simulink model "Open_Loop_No_PLL"  (R2020b)
settings: Solver=ode1  StartTime=0  StopTime=1  FixedStep=Time_Step  MaxStep=100e-6  RelTol=1e-3
undefined symbols (not defined in the file): fb, fn, Ib2, Kp_Rvi_pu, Lc_eq, Lg, Rg, Sb, SCR, Sn, Theta_Vvsc0, Time_Step, Va0, Vb0, Vb1, Vb2, Vc0, Vm0, VSC01_id0, Vvsc0, wb, Zb
libraries: powerlib x23, Control_Lib x22, Source_Lib x3, simulink x2
(part 2 of 2)

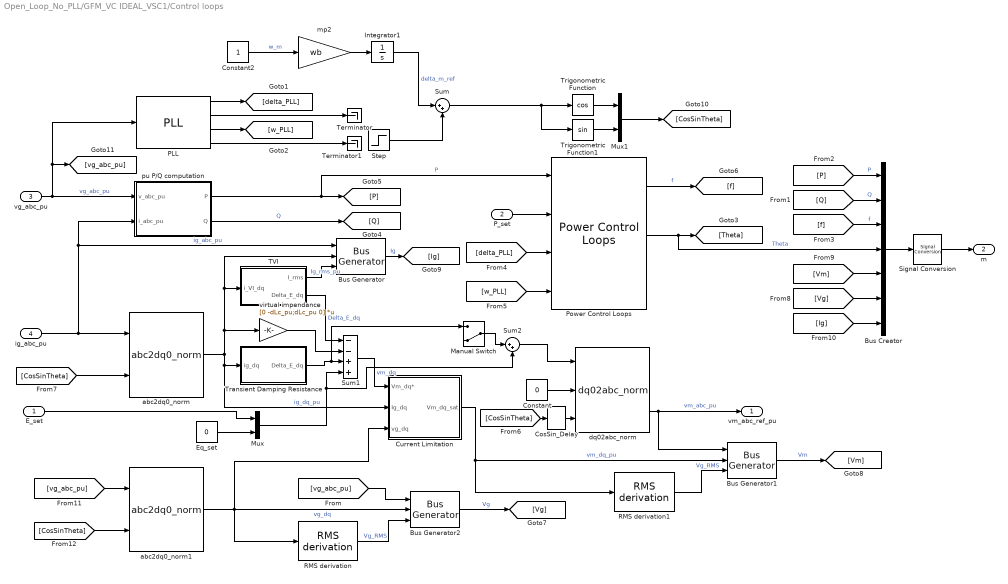
== system Open_Loop_No_PLL/GFM_VC IDEAL_VSC1/Control loops ==
  E_set : Inport
  P_set : Inport  Port=2
  vg_abc_pu : Inport  Port=3
  ig_abc_pu : Inport  Port=4
  " pu P/Q computation" : Subsystem  DialogController=POWERSYS.PowerSysDialog
  Bus Creator : BusCreator  Inputs=7
  Bus Generator : Control_Lib/Bus Generator  Gpu=Ib2
      settings: SourceProductName=VSC4SPS
  Bus Generator1 : Control_Lib/Bus Generator  Gpu=Vb1
      settings: SourceProductName=VSC4SPS
  Bus Generator2 : Control_Lib/Bus Generator  Gpu=Vb2
      settings: SourceProductName=VSC4SPS
  Constant : Constant  Value=0
  Constant2 : Constant
  CosSin_Delay : Control_Lib/CosSin_Delay  dTheta=wb*(Output_Delay)
      settings: SourceProductName=VSC4SPS
  Current Limitation : Subsystem
  Eq_set : Constant  Value=0
  Integrator1 : Integrator  InitialCondition=Theta_Vvsc0*pi/180
  Manual Switch : ManualSwitch  CurrentSetting=0
  Mux : Mux  Inputs=2
  Mux1 : Mux  Inputs=[1 1]
  PLL : Control_Lib/PLL  fb=fb  wn_PLL=wn_PLL  zeta_PLL=zeta_PLL  Theta0=Theta0
      settings: SourceProductName=VSC4SPS
  Power Control Loops : Control_Lib/Power Control Loops  Theta0_VSC=Theta_Vvsc0
      settings: SourceProductName=VSC4SPS
  RMS derivation : Control_Lib/RMS derivation  SystemSampleTime=-1  VariantActivationTime=update diagram  Latency=0  AutoFrameSizeCalculation=off
      settings: SourceProductName=VSC4SPS
  RMS derivation1 : Control_Lib/RMS derivation  SystemSampleTime=-1  VariantActivationTime=update diagram  Latency=0  AutoFrameSizeCalculation=off
      settings: SourceProductName=VSC4SPS
  Signal Conversion : SignalConversion  OverrideOpt=off
  Step : Step  Time=0.2  After=asin(0.5*(Lc_eq+1/SCR))  SampleTime=0
  Sum : Sum  Inputs=|++
  Sum1 : Sum  Inputs=--++
  Sum2 : Sum  Inputs=|++
  TVI : Subsystem
  Terminator : Terminator
  Terminator1 : Terminator
  Transient Damping Resistance : Subsystem
  Trigonometric Function : Trigonometry  Operator=cos
  Trigonometric Function1 : Trigonometry
  abc2dq0_norm : Control_Lib/abc2dq0_norm  referenceAxisMode=Reference axis at 90 degrees behind phase_a  baseUpdateGain=1/sqrt(3)
      settings: SourceProductName=VSC4SPS
  abc2dq0_norm1 : Control_Lib/abc2dq0_norm  referenceAxisMode=Reference axis at 90 degrees behind phase_a  baseUpdateGain=1/sqrt(3)
      settings: SourceProductName=VSC4SPS
  dq02abc_norm : Control_Lib/dq02abc_norm  referenceAxisMode=Reference axis at 90 degrees behind phase_a  baseUpdateGain=sqrt(3)
      settings: SourceProductName=VSC4SPS
  mp2 : Gain  Gain=wb
  virtual impendance : Gain  Gain=[0 -dLc_pu;dLc_pu 0]  Multiplication=Matrix(K*u)
  vm_abc_ref_pu : Outport  VectorParamsAs1DForOutWhenUnconnected=off
  m : Outport  Port=2  VectorParamsAs1DForOutWhenUnconnected=off
  wires:
  virtual impendance/1 -> Sum1/2
  [Vg] -> Bus Creator/6
  Bus Generator2/1 -> [Vg]  "Vg"
  [Ig] -> Bus Creator/7
  RMS derivation1/1 -> Bus Generator1/3  "Vg_RMS"
  Bus Generator1/1 -> [Vm]  "Vm"
  TVI/1(I_rms) -> Bus Generator/3  "Ig_rms_pu"
  RMS derivation/1 -> Bus Generator2/3  "Vg_RMS"
  Signal Conversion/1 -> m/1
  [P] -> Bus Creator/1  "P"
  [Q] -> Bus Creator/2  "Q"
  [f] -> Bus Creator/3  "f"
  dq02abc_norm/2 -> vm_abc_ref_pu/1, Bus Generator1/1  "vm_abc_pu"
  E_set/1 -> Mux/1
  " pu P/Q computation"/2(Q) -> [Q]  "Q"
  Current Limitation/1(Vm_dq_sat) -> Bus Generator1/2, RMS derivation1/1  "vm_dq_pu"
  [delta_PLL] -> Power Control Loops/3
  P_set/1 -> Power Control Loops/2
  [w_PLL] -> Power Control Loops/4
  Power Control Loops/1 -> [f]  "f"
  vg_abc_pu/1 -> " pu P/Q computation"/1(v_abc_pu), [vg_abc_pu], PLL/1  "vg_abc_pu"
  " pu P/Q computation"/1(P) -> Power Control Loops/1, [P]  "P"
  ig_abc_pu/1 -> " pu P/Q computation"/2(i_abc_pu), Bus Generator/1, abc2dq0_norm/1  "ig_abc_pu"
  abc2dq0_norm/2 -> virtual impendance/1, TVI/1(i_VI_dq), Bus Generator/2, Transient Damping Resistance/1(ig_dq), Current Limitation/2(Ig_dq)  "ig_dq_pu"
  Power Control Loops/2 -> [Theta], Bus Creator/4  "Theta"
  [CosSinTheta] -> abc2dq0_norm/2
  TVI/2(Delta_E_dq) -> Sum1/1  "Delta_E_dq"
  Transient Damping Resistance/1("Delta_E_dq ") -> Manual Switch/1, Sum1/3
  Mux/1 -> Sum2/2, Sum1/4
  Eq_set/1 -> Mux/2
  [Vm] -> Bus Creator/5
  Bus Creator/1 -> Signal Conversion/1
  Bus Generator/1 -> [Ig]  "Ig"
  PLL/3 -> [w_PLL]
  Constant/1 -> dq02abc_norm/2
  PLL/1 -> [delta_PLL]
  PLL/2 -> Terminator/1
  PLL/4 -> Terminator1/1
  [vg_abc_pu] -> Bus Generator2/1
  Sum1/1 -> Current Limitation/1(Vm_dq*)  "vm_dq"
  abc2dq0_norm1/2 -> Bus Generator2/2, Current Limitation/3(vg_dq), RMS derivation/1  "vg_dq"
  [vg_abc_pu] -> abc2dq0_norm1/1
  [CosSinTheta] -> abc2dq0_norm1/2
  [CosSinTheta] -> CosSin_Delay/1
  CosSin_Delay/1 -> dq02abc_norm/3
  Step/1 -> Sum/2
  Trigonometric Function/1 -> Mux1/1
  Mux1/1 -> [CosSinTheta]
  Trigonometric Function1/1 -> Mux1/2
  Sum/1 -> Trigonometric Function1/1, Trigonometric Function/1
  Manual Switch/1 -> Sum2/1
  Sum2/1 -> dq02abc_norm/1
  Integrator1/1 -> Sum/1  "delta_m_ref"
  Constant2/1 -> mp2/1  "w_m"
  mp2/1 -> Integrator1/1

== system Open_Loop_No_PLL/GFM_VC IDEAL_VSC/Control loops/ pu P//Q computation ==
  v_abc_pu : Inport  PortDimensions=3
  i_abc_pu : Inport  Port=2  PortDimensions=3
  Demux : Demux  Outputs=3
      settings: DisplayOption=none
  Mux : Mux  Inputs=3
  Product1 : Product  InputSameDT=on  SaturateOnIntegerOverflow=on  OutDataTypeStr=Inherit: Same as first input
  Product3 : Product  InputSameDT=on  SaturateOnIntegerOverflow=on  OutDataTypeStr=Inherit: Same as first input
  Sum : Sum  Inputs=+-  InputSameDT=on  SaturateOnIntegerOverflow=on  OutDataTypeStr=Inherit: Same as first input
  Sum1 : Sum  Inputs=1  InputSameDT=on  SaturateOnIntegerOverflow=on  OutDataTypeStr=Inherit: Same as first input
  Sum4 : Sum  Inputs=1  InputSameDT=on  SaturateOnIntegerOverflow=on  OutDataTypeStr=Inherit: Same as first input
  Sum5 : Sum  Inputs=+-  InputSameDT=on  SaturateOnIntegerOverflow=on  OutDataTypeStr=Inherit: Same as first input
  Sum6 : Sum  Inputs=+-  InputSameDT=on  SaturateOnIntegerOverflow=on  OutDataTypeStr=Inherit: Same as first input
  pu->V : Gain  Gain=1/sqrt(3)  SaturateOnIntegerOverflow=on  OutDataTypeStr=Inherit: Same as input  ParamDataTypeStr=Inherit: Same as input
  pu->V1 : Gain  Gain=1/3  SaturateOnIntegerOverflow=on  OutDataTypeStr=Inherit: Same as input  ParamDataTypeStr=Inherit: Same as input
  pu->V2 : Gain  Gain=1/3  SaturateOnIntegerOverflow=on  OutDataTypeStr=Inherit: Same as input  ParamDataTypeStr=Inherit: Same as input
  P : Outport  VectorParamsAs1DForOutWhenUnconnected=off
  Q : Outport  Port=2  VectorParamsAs1DForOutWhenUnconnected=off
  wires:
  pu->V/1 -> pu->V2/1  "Q"
  Mux/1 -> Product3/1
  Sum6/1 -> Mux/2
  Sum5/1 -> Mux/1
  Sum/1 -> Mux/3
  Demux/3 -> Sum6/1, Sum5/2
  Demux/2 -> Sum5/1, Sum/2
  Demux/1 -> Sum6/2, Sum/1
  Sum4/1 -> pu->V1/1
  i_abc_pu/1 -> Product3/2, Product1/2
  v_abc_pu/1 -> Demux/1, Product1/1
  Product1/1 -> Sum4/1
  Product3/1 -> Sum1/1
  Sum1/1 -> pu->V/1
  pu->V1/1 -> P/1
  pu->V2/1 -> Q/1

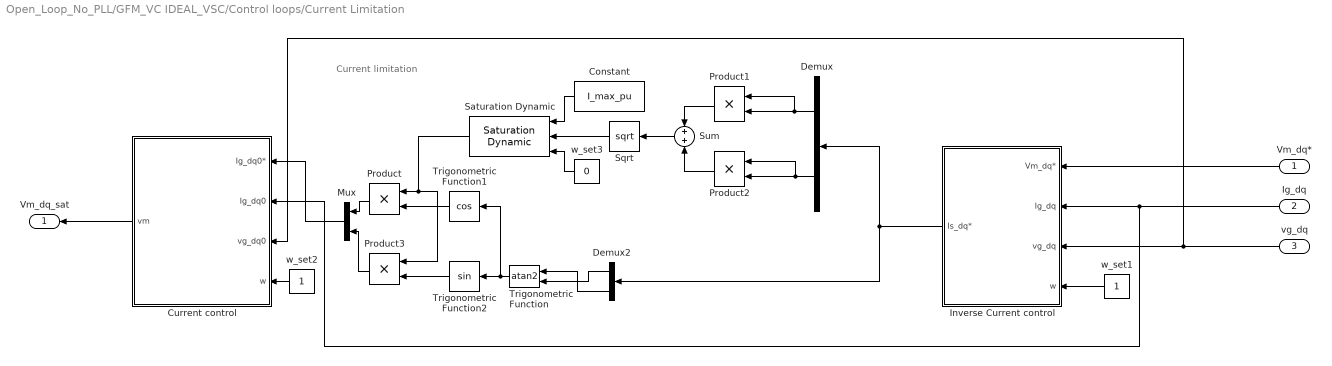
== system Open_Loop_No_PLL/GFM_VC IDEAL_VSC/Control loops/Current Limitation ==
  note: Current limitation
  Vm_dq* : Inport
  Ig_dq : Inport  Port=2
  vg_dq : Inport  Port=3
  Constant : Constant  Value=I_max_pu
  Current control : Subsystem
  Demux : Demux  Outputs=2
  Demux2 : Demux  Outputs=2
  Inverse Current control : Subsystem
  Mux : Mux  Inputs=2
  Product{,1..3} (4 alike) : Product
  Saturation Dynamic : simulink/Discontinuities/Saturation Dynamic  OutMin=[]  OutMax=[]  OutDataTypeStr=Inherit: Same as second input  OutDataType=fixdt(1, 16)  OutScaling=2^-10  DoSatur=off
  Sqrt : Sqrt  SaturateOnIntegerOverflow=on
  Sum : Sum
  Trigonometric Function : Trigonometry  Operator=atan2  NumberOfIterations=5  OutputSignalType=real
  Trigonometric Function1 : Trigonometry  Operator=cos
  Trigonometric Function2 : Trigonometry
  w_set1 : Constant
  w_set2 : Constant
  w_set3 : Constant  Value=0
  Vm_dq_sat : Outport  VectorParamsAs1DForOutWhenUnconnected=off
  wires:
  Current control/1(vm) -> Vm_dq_sat/1
  Vm_dq*/1 -> Inverse Current control/1(Vm_dq*)
  vg_dq/1 -> Inverse Current control/3(vg_dq), Current control/3(vg_dq0)
  w_set2/1 -> Current control/4(w)
  w_set1/1 -> Inverse Current control/4(w)
  Ig_dq/1 -> Current control/2(Ig_dq0), Inverse Current control/2(Ig_dq)
  Product3/1 -> Mux/2
  Sum/1 -> Sqrt/1
  Inverse Current control/1(Is_dq*) -> Demux/1, Demux2/1
  Demux2/2 -> Trigonometric Function/1
  Sqrt/1 -> Saturation Dynamic/2
  Product1/1 -> Sum/1
  Saturation Dynamic/1 -> Product3/1, Product/1
  Trigonometric Function/1 -> Trigonometric Function1/1, Trigonometric Function2/1
  Demux2/1 -> Trigonometric Function/2
  Trigonometric Function1/1 -> Product/2
  Product2/1 -> Sum/2
  Trigonometric Function2/1 -> Product3/2
  Demux/2 -> Product2/2, Product2/1
  Demux/1 -> Product1/2, Product1/1
  Product/1 -> Mux/1
  Mux/1 -> Current control/1(Ig_dq0*)
  Constant/1 -> Saturation Dynamic/1
  w_set3/1 -> Saturation Dynamic/3

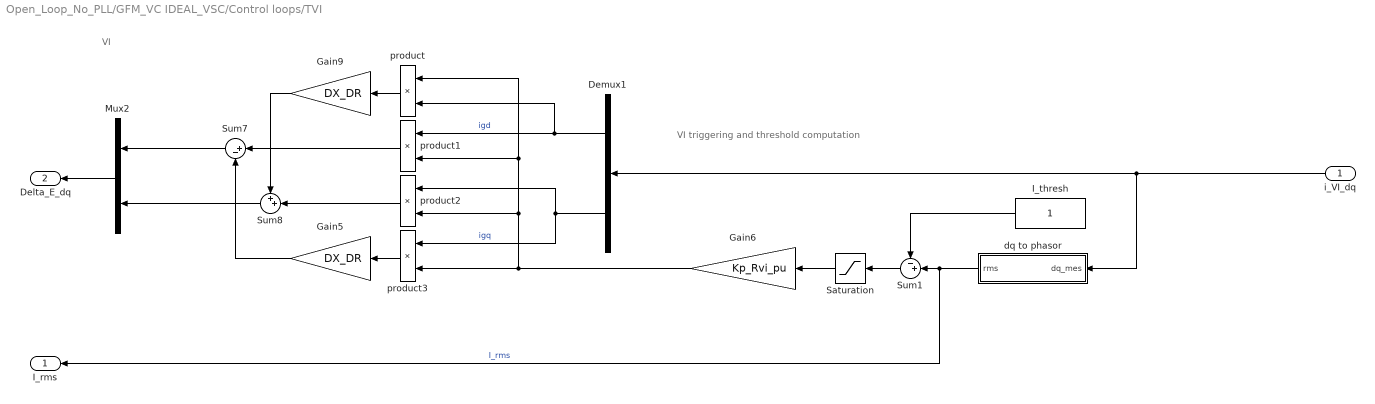
== system Open_Loop_No_PLL/GFM_VC IDEAL_VSC/Control loops/TVI ==
  note: VI
  note: VI triggering and threshold computation
  i_VI_dq : Inport
  Demux1 : Demux  Outputs=2
      settings: DisplayOption=none
  Gain5 : Gain  Gain=DX_DR
  Gain6 : Gain  Gain=Kp_Rvi_pu
  Gain9 : Gain  Gain=DX_DR
  I_thresh : Constant
  Mux2 : Mux  Inputs=2
  Saturation : Saturate  UpperLimit=inf  LowerLimit=0
  Sum1 : Sum  Inputs=-+|
  Sum7 : Sum  Inputs=|+-
  Sum8 : Sum  Inputs=++|
  dq to phasor : Subsystem
  product{,1..3} (4 alike) : Product  InputSameDT=on  RndMeth=Zero  SaturateOnIntegerOverflow=on  OutDataTypeStr=Inherit: Same as first input
  I_rms : Outport  VectorParamsAs1DForOutWhenUnconnected=off
  Delta_E_dq : Outport  Port=2  VectorParamsAs1DForOutWhenUnconnected=off
  wires:
  i_VI_dq/1 -> Demux1/1, dq to phasor/1(dq_mes)
  Sum8/1 -> Mux2/2
  Sum7/1 -> Mux2/1
  product2/1 -> Sum8/2
  Gain9/1 -> Sum8/1
  Gain5/1 -> Sum7/2
  product1/1 -> Sum7/1
  Demux1/2 -> product3/1, product2/1  "igq"
  Demux1/1 -> product/2, product1/1  "igd"
  product/1 -> Gain9/1
  product3/1 -> Gain5/1
  Gain6/1 -> product2/2, product1/2, product/1, product3/2
  Mux2/1 -> Delta_E_dq/1
  I_thresh/1 -> Sum1/1
  Saturation/1 -> Gain6/1
  dq to phasor/1(rms) -> I_rms/1, Sum1/2  "I_rms"
  Sum1/1 -> Saturation/1

== system Open_Loop_No_PLL/GFM_VC IDEAL_VSC/Control loops/Transient Damping Resistance ==
  ig_dq : Inport
  Filter w_LF : Subsystem
      mask Display: disp('\omega_{LF} / (s + \omega_{LF})','texmode','on')
  Sum5 : Sum  Inputs=|+-
  nq1 : Gain  Gain=Rv
  "Delta_E_dq " : Outport  VectorParamsAs1DForOutWhenUnconnected=off
  wires:
  ig_dq/1 -> nq1/1
  Sum5/1 -> "Delta_E_dq "/1
  Filter w_LF/1(s) -> Sum5/1
  nq1/1 -> Sum5/2, Filter w_LF/1(e)

== system Open_Loop_No_PLL/GFM_VC IDEAL_VSC1/Control loops/ pu P//Q computation ==
  v_abc_pu : Inport  PortDimensions=3
  i_abc_pu : Inport  Port=2  PortDimensions=3
  Demux : Demux  Outputs=3
      settings: DisplayOption=none
  Mux : Mux  Inputs=3
  Product1 : Product  InputSameDT=on  SaturateOnIntegerOverflow=on  OutDataTypeStr=Inherit: Same as first input
  Product3 : Product  InputSameDT=on  SaturateOnIntegerOverflow=on  OutDataTypeStr=Inherit: Same as first input
  Sum : Sum  Inputs=+-  InputSameDT=on  SaturateOnIntegerOverflow=on  OutDataTypeStr=Inherit: Same as first input
  Sum1 : Sum  Inputs=1  InputSameDT=on  SaturateOnIntegerOverflow=on  OutDataTypeStr=Inherit: Same as first input
  Sum4 : Sum  Inputs=1  InputSameDT=on  SaturateOnIntegerOverflow=on  OutDataTypeStr=Inherit: Same as first input
  Sum5 : Sum  Inputs=+-  InputSameDT=on  SaturateOnIntegerOverflow=on  OutDataTypeStr=Inherit: Same as first input
  Sum6 : Sum  Inputs=+-  InputSameDT=on  SaturateOnIntegerOverflow=on  OutDataTypeStr=Inherit: Same as first input
  pu->V : Gain  Gain=1/sqrt(3)  SaturateOnIntegerOverflow=on  OutDataTypeStr=Inherit: Same as input  ParamDataTypeStr=Inherit: Same as input
  pu->V1 : Gain  Gain=1/3  SaturateOnIntegerOverflow=on  OutDataTypeStr=Inherit: Same as input  ParamDataTypeStr=Inherit: Same as input
  pu->V2 : Gain  Gain=1/3  SaturateOnIntegerOverflow=on  OutDataTypeStr=Inherit: Same as input  ParamDataTypeStr=Inherit: Same as input
  P : Outport  VectorParamsAs1DForOutWhenUnconnected=off
  Q : Outport  Port=2  VectorParamsAs1DForOutWhenUnconnected=off
  wires:
  pu->V/1 -> pu->V2/1  "Q"
  Mux/1 -> Product3/1
  Sum6/1 -> Mux/2
  Sum5/1 -> Mux/1
  Sum/1 -> Mux/3
  Demux/3 -> Sum6/1, Sum5/2
  Demux/2 -> Sum5/1, Sum/2
  Demux/1 -> Sum6/2, Sum/1
  Sum4/1 -> pu->V1/1
  i_abc_pu/1 -> Product3/2, Product1/2
  v_abc_pu/1 -> Demux/1, Product1/1
  Product1/1 -> Sum4/1
  Product3/1 -> Sum1/1
  Sum1/1 -> pu->V/1
  pu->V1/1 -> P/1
  pu->V2/1 -> Q/1

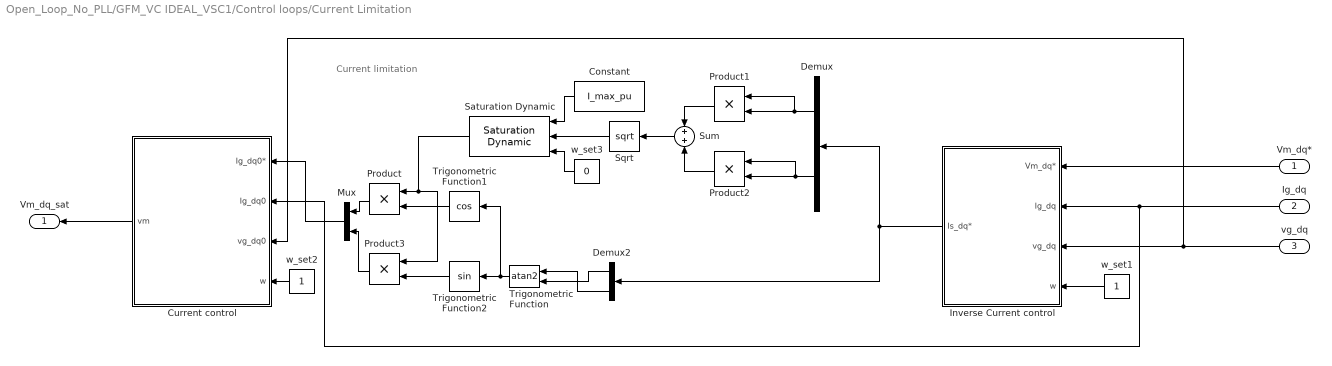
== system Open_Loop_No_PLL/GFM_VC IDEAL_VSC1/Control loops/Current Limitation ==
  note: Current limitation
  Vm_dq* : Inport
  Ig_dq : Inport  Port=2
  vg_dq : Inport  Port=3
  Constant : Constant  Value=I_max_pu
  Current control : Subsystem
  Demux : Demux  Outputs=2
  Demux2 : Demux  Outputs=2
  Inverse Current control : Subsystem
  Mux : Mux  Inputs=2
  Product{,1..3} (4 alike) : Product
  Saturation Dynamic : simulink/Discontinuities/Saturation Dynamic  OutMin=[]  OutMax=[]  OutDataTypeStr=Inherit: Same as second input  OutDataType=fixdt(1, 16)  OutScaling=2^-10  DoSatur=off
  Sqrt : Sqrt  SaturateOnIntegerOverflow=on
  Sum : Sum
  Trigonometric Function : Trigonometry  Operator=atan2  NumberOfIterations=5  OutputSignalType=real
  Trigonometric Function1 : Trigonometry  Operator=cos
  Trigonometric Function2 : Trigonometry
  w_set1 : Constant
  w_set2 : Constant
  w_set3 : Constant  Value=0
  Vm_dq_sat : Outport  VectorParamsAs1DForOutWhenUnconnected=off
  wires:
  Current control/1(vm) -> Vm_dq_sat/1
  Vm_dq*/1 -> Inverse Current control/1(Vm_dq*)
  vg_dq/1 -> Inverse Current control/3(vg_dq), Current control/3(vg_dq0)
  w_set2/1 -> Current control/4(w)
  w_set1/1 -> Inverse Current control/4(w)
  Ig_dq/1 -> Current control/2(Ig_dq0), Inverse Current control/2(Ig_dq)
  Product3/1 -> Mux/2
  Sum/1 -> Sqrt/1
  Inverse Current control/1(Is_dq*) -> Demux/1, Demux2/1
  Demux2/2 -> Trigonometric Function/1
  Sqrt/1 -> Saturation Dynamic/2
  Product1/1 -> Sum/1
  Saturation Dynamic/1 -> Product3/1, Product/1
  Trigonometric Function/1 -> Trigonometric Function1/1, Trigonometric Function2/1
  Demux2/1 -> Trigonometric Function/2
  Trigonometric Function1/1 -> Product/2
  Product2/1 -> Sum/2
  Trigonometric Function2/1 -> Product3/2
  Demux/2 -> Product2/2, Product2/1
  Demux/1 -> Product1/2, Product1/1
  Product/1 -> Mux/1
  Mux/1 -> Current control/1(Ig_dq0*)
  Constant/1 -> Saturation Dynamic/1
  w_set3/1 -> Saturation Dynamic/3

== system Open_Loop_No_PLL/GFM_VC IDEAL_VSC1/Control loops/TVI ==
  note: VI
  note: VI triggering and threshold computation
  i_VI_dq : Inport
  Demux1 : Demux  Outputs=2
      settings: DisplayOption=none
  Gain5 : Gain  Gain=DX_DR
  Gain6 : Gain  Gain=Kp_Rvi_pu
  Gain9 : Gain  Gain=DX_DR
  I_thresh : Constant
  Mux2 : Mux  Inputs=2
  Saturation : Saturate  UpperLimit=inf  LowerLimit=0
  Sum1 : Sum  Inputs=-+|
  Sum7 : Sum  Inputs=|+-
  Sum8 : Sum  Inputs=++|
  dq to phasor : Subsystem
  product{,1..3} (4 alike) : Product  InputSameDT=on  RndMeth=Zero  SaturateOnIntegerOverflow=on  OutDataTypeStr=Inherit: Same as first input
  I_rms : Outport  VectorParamsAs1DForOutWhenUnconnected=off
  Delta_E_dq : Outport  Port=2  VectorParamsAs1DForOutWhenUnconnected=off
  wires:
  i_VI_dq/1 -> Demux1/1, dq to phasor/1(dq_mes)
  Sum8/1 -> Mux2/2
  Sum7/1 -> Mux2/1
  product2/1 -> Sum8/2
  Gain9/1 -> Sum8/1
  Gain5/1 -> Sum7/2
  product1/1 -> Sum7/1
  Demux1/2 -> product3/1, product2/1  "igq"
  Demux1/1 -> product/2, product1/1  "igd"
  product/1 -> Gain9/1
  product3/1 -> Gain5/1
  Gain6/1 -> product2/2, product1/2, product/1, product3/2
  Mux2/1 -> Delta_E_dq/1
  I_thresh/1 -> Sum1/1
  Saturation/1 -> Gain6/1
  dq to phasor/1(rms) -> I_rms/1, Sum1/2  "I_rms"
  Sum1/1 -> Saturation/1

== system Open_Loop_No_PLL/GFM_VC IDEAL_VSC1/Control loops/Transient Damping Resistance ==
  ig_dq : Inport
  Filter w_LF : Subsystem
      mask Display: disp('\omega_{LF} / (s + \omega_{LF})','texmode','on')
  Sum5 : Sum  Inputs=|+-
  nq1 : Gain  Gain=Rv
  "Delta_E_dq " : Outport  VectorParamsAs1DForOutWhenUnconnected=off
  wires:
  ig_dq/1 -> nq1/1
  Sum5/1 -> "Delta_E_dq "/1
  Filter w_LF/1(s) -> Sum5/1
  nq1/1 -> Sum5/2, Filter w_LF/1(e)

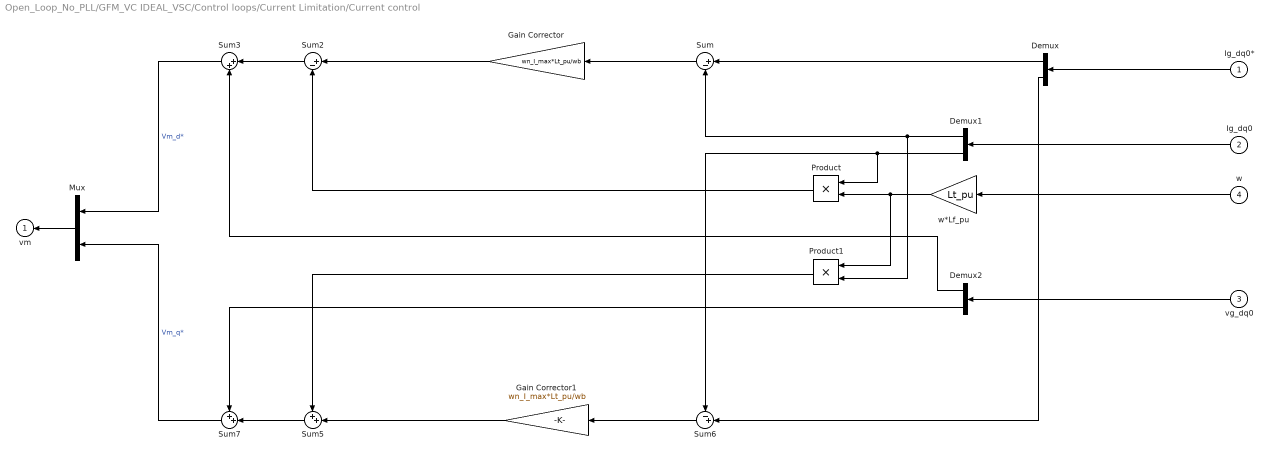
== system Open_Loop_No_PLL/GFM_VC IDEAL_VSC/Control loops/Current Limitation/Current control ==
  Ig_dq0* : Inport
  Ig_dq0 : Inport  Port=2
  vg_dq0 : Inport  Port=3
  w : Inport  Port=4
  Demux : Demux  Outputs=2
  Demux1 : Demux  Outputs=2
  Demux2 : Demux  Outputs=2
  Gain Corrector : Gain  Gain=wn_I_max*Lt_pu/wb
  Gain Corrector1 : Gain  Gain=wn_I_max*Lt_pu/wb
  Mux : Mux  Inputs=2
  Product : Product  RndMeth=Zero
  Product1 : Product  RndMeth=Zero
  Sum : Sum  Inputs=|+-
  Sum2 : Sum  Inputs=|+-
  Sum3 : Sum  Inputs=|++
  Sum5 : Sum  Inputs=++|
  Sum6 : Sum  Inputs=-+|
  Sum7 : Sum  Inputs=++|
  w*Lf_pu : Gain  Gain=Lt_pu
  vm : Outport  InitialOutput=0  VectorParamsAs1DForOutWhenUnconnected=off
  wires:
  Mux/1 -> vm/1
  Ig_dq0*/1 -> Demux/1
  Sum6/1 -> Gain Corrector1/1
  vg_dq0/1 -> Demux2/1
  Ig_dq0/1 -> Demux1/1
  Demux/1 -> Sum/1
  Demux1/1 -> Product1/2, Sum/2
  Gain Corrector/1 -> Sum2/1
  w*Lf_pu/1 -> Product1/1, Product/2
  Demux1/2 -> Product/1, Sum6/1
  Product/1 -> Sum2/2
  Sum2/1 -> Sum3/1
  Demux/2 -> Sum6/2
  Gain Corrector1/1 -> Sum5/2
  Product1/1 -> Sum5/1
  Sum5/1 -> Sum7/2
  Sum3/1 -> Mux/1  "Vm_d*"
  Sum7/1 -> Mux/2  "Vm_q*"
  Sum/1 -> Gain Corrector/1
  w/1 -> w*Lf_pu/1
  Demux2/1 -> Sum3/2
  Demux2/2 -> Sum7/1

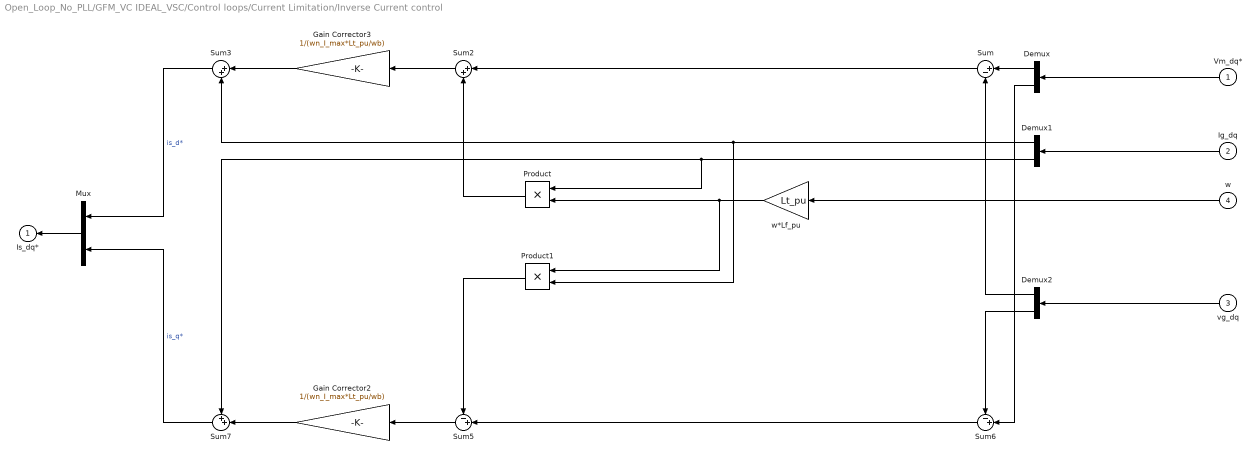
== system Open_Loop_No_PLL/GFM_VC IDEAL_VSC/Control loops/Current Limitation/Inverse Current control ==
  Vm_dq* : Inport
  Ig_dq : Inport  Port=2
  vg_dq : Inport  Port=3
  w : Inport  Port=4
  Demux : Demux  Outputs=2
  Demux1 : Demux  Outputs=2
  Demux2 : Demux  Outputs=2
  Gain Corrector2 : Gain  Gain=1/(wn_I_max*Lt_pu/wb)
  Gain Corrector3 : Gain  Gain=1/(wn_I_max*Lt_pu/wb)
  Mux : Mux  Inputs=2
  Product : Product  RndMeth=Zero
  Product1 : Product  RndMeth=Zero
  Sum : Sum  Inputs=|+-
  Sum2 : Sum  Inputs=|++
  Sum3 : Sum  Inputs=|++
  Sum5 : Sum  Inputs=-+|
  Sum6 : Sum  Inputs=-+|
  Sum7 : Sum  Inputs=++|
  w*Lf_pu : Gain  Gain=Lt_pu
  Is_dq* : Outport  InitialOutput=0  VectorParamsAs1DForOutWhenUnconnected=off
  wires:
  Gain Corrector2/1 -> Sum7/2
  Product1/1 -> Sum5/1
  Demux2/2 -> Sum6/1
  Demux2/1 -> Sum/2
  Gain Corrector3/1 -> Sum3/1
  Demux1/2 -> Product/1, Sum7/1
  w/1 -> w*Lf_pu/1
  Sum7/1 -> Mux/2  "is_q*"
  Sum3/1 -> Mux/1  "is_d*"
  Sum5/1 -> Gain Corrector2/1
  Sum6/1 -> Sum5/2
  Demux/2 -> Sum6/2
  Mux/1 -> Is_dq*/1
  Sum2/1 -> Gain Corrector3/1
  Product/1 -> Sum2/2
  w*Lf_pu/1 -> Product/2, Product1/1
  Sum/1 -> Sum2/1
  Demux1/1 -> Product1/2, Sum3/2
  Demux/1 -> Sum/1
  Vm_dq*/1 -> Demux/1
  Ig_dq/1 -> Demux1/1
  vg_dq/1 -> Demux2/1

== system Open_Loop_No_PLL/GFM_VC IDEAL_VSC/Control loops/TVI/dq to phasor ==
  dq_mes : Inport
  Demux : Demux  Outputs=2
      settings: DisplayOption=none
  Sqrt : Sqrt  SaturateOnIntegerOverflow=on
  Sum4 : Sum  Inputs=|++  InputSameDT=on  SaturateOnIntegerOverflow=on  OutDataTypeStr=Inherit: Same as first input
  Vrdird : Product  InputSameDT=on  RndMeth=Zero  SaturateOnIntegerOverflow=on  OutDataTypeStr=Inherit: Same as first input
  Vrqirq : Product  InputSameDT=on  RndMeth=Zero  SaturateOnIntegerOverflow=on  OutDataTypeStr=Inherit: Same as first input
  rms : Outport  VectorParamsAs1DForOutWhenUnconnected=off
  wires:
  Sqrt/1 -> rms/1
  dq_mes/1 -> Demux/1
  Demux/1 -> Vrdird/1, Vrdird/2
  Demux/2 -> Vrqirq/1, Vrqirq/2
  Vrdird/1 -> Sum4/1
  Vrqirq/1 -> Sum4/2
  Sum4/1 -> Sqrt/1

== system Open_Loop_No_PLL/GFM_VC IDEAL_VSC/Control loops/Transient Damping Resistance/Filter w_LF ==
  e : Inport
  1/T_LP : Gain  Gain=W_TVR  SaturateOnIntegerOverflow=on  OutDataTypeStr=Inherit: Same as input  ParamDataTypeStr=Inherit: Same as input
  Integrator : Integrator  InitialConditionSource=external  InitialCondition=[VSC01_id0*0.04]
  Sum1 : Sum  Inputs=|+-  InputSameDT=on  SaturateOnIntegerOverflow=on  OutDataTypeStr=Inherit: Same as first input
  s : Outport  VectorParamsAs1DForOutWhenUnconnected=off
  wires:
  Sum1/1 -> 1/T_LP/1
  1/T_LP/1 -> Integrator/1
  Integrator/1 -> Sum1/2, s/1
  e/1 -> Integrator/2, Sum1/1

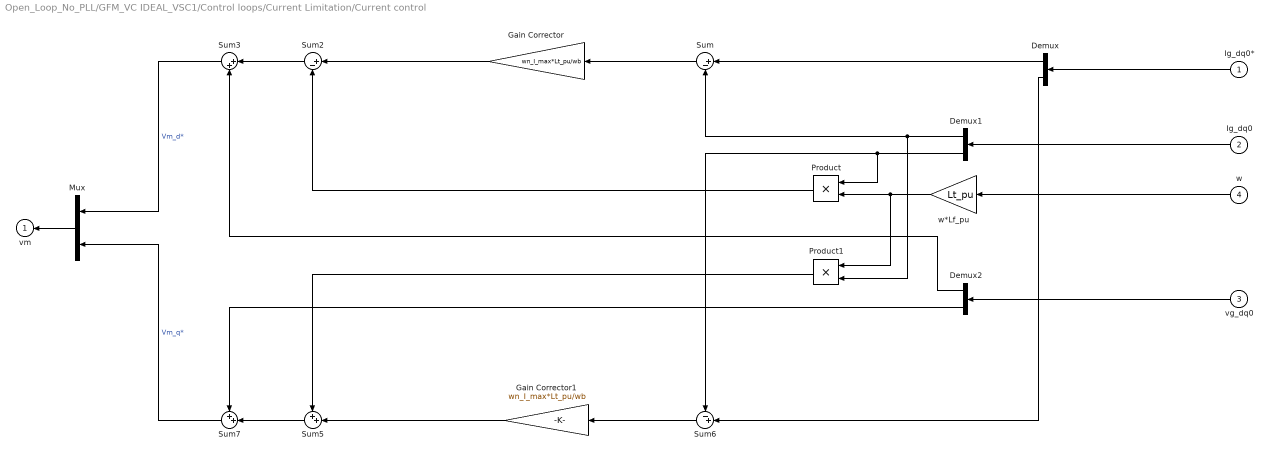
== system Open_Loop_No_PLL/GFM_VC IDEAL_VSC1/Control loops/Current Limitation/Current control ==
  Ig_dq0* : Inport
  Ig_dq0 : Inport  Port=2
  vg_dq0 : Inport  Port=3
  w : Inport  Port=4
  Demux : Demux  Outputs=2
  Demux1 : Demux  Outputs=2
  Demux2 : Demux  Outputs=2
  Gain Corrector : Gain  Gain=wn_I_max*Lt_pu/wb
  Gain Corrector1 : Gain  Gain=wn_I_max*Lt_pu/wb
  Mux : Mux  Inputs=2
  Product : Product  RndMeth=Zero
  Product1 : Product  RndMeth=Zero
  Sum : Sum  Inputs=|+-
  Sum2 : Sum  Inputs=|+-
  Sum3 : Sum  Inputs=|++
  Sum5 : Sum  Inputs=++|
  Sum6 : Sum  Inputs=-+|
  Sum7 : Sum  Inputs=++|
  w*Lf_pu : Gain  Gain=Lt_pu
  vm : Outport  InitialOutput=0  VectorParamsAs1DForOutWhenUnconnected=off
  wires:
  Mux/1 -> vm/1
  Ig_dq0*/1 -> Demux/1
  Sum6/1 -> Gain Corrector1/1
  vg_dq0/1 -> Demux2/1
  Ig_dq0/1 -> Demux1/1
  Demux/1 -> Sum/1
  Demux1/1 -> Product1/2, Sum/2
  Gain Corrector/1 -> Sum2/1
  w*Lf_pu/1 -> Product1/1, Product/2
  Demux1/2 -> Product/1, Sum6/1
  Product/1 -> Sum2/2
  Sum2/1 -> Sum3/1
  Demux/2 -> Sum6/2
  Gain Corrector1/1 -> Sum5/2
  Product1/1 -> Sum5/1
  Sum5/1 -> Sum7/2
  Sum3/1 -> Mux/1  "Vm_d*"
  Sum7/1 -> Mux/2  "Vm_q*"
  Sum/1 -> Gain Corrector/1
  w/1 -> w*Lf_pu/1
  Demux2/1 -> Sum3/2
  Demux2/2 -> Sum7/1

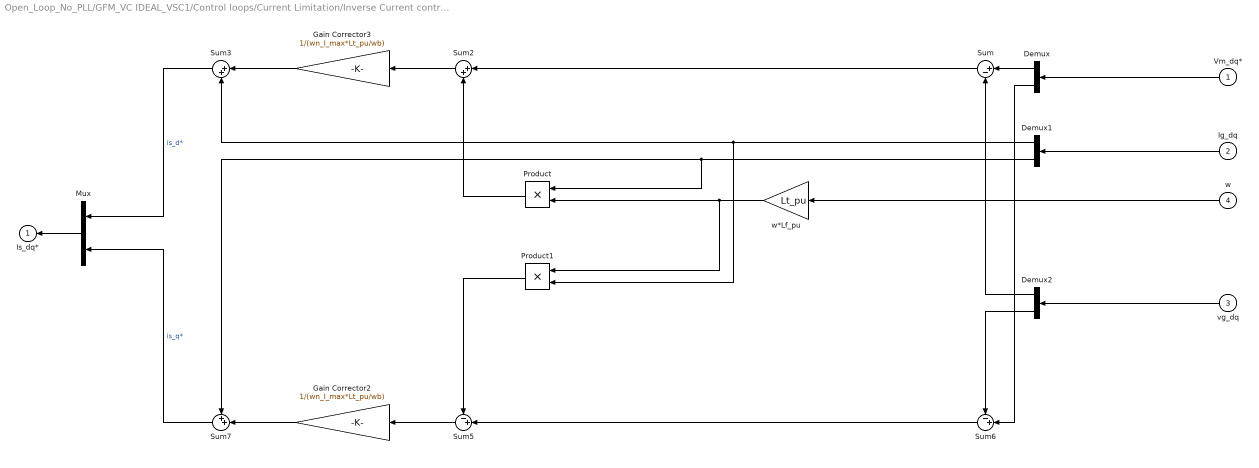
== system Open_Loop_No_PLL/GFM_VC IDEAL_VSC1/Control loops/Current Limitation/Inverse Current control ==
  Vm_dq* : Inport
  Ig_dq : Inport  Port=2
  vg_dq : Inport  Port=3
  w : Inport  Port=4
  Demux : Demux  Outputs=2
  Demux1 : Demux  Outputs=2
  Demux2 : Demux  Outputs=2
  Gain Corrector2 : Gain  Gain=1/(wn_I_max*Lt_pu/wb)
  Gain Corrector3 : Gain  Gain=1/(wn_I_max*Lt_pu/wb)
  Mux : Mux  Inputs=2
  Product : Product  RndMeth=Zero
  Product1 : Product  RndMeth=Zero
  Sum : Sum  Inputs=|+-
  Sum2 : Sum  Inputs=|++
  Sum3 : Sum  Inputs=|++
  Sum5 : Sum  Inputs=-+|
  Sum6 : Sum  Inputs=-+|
  Sum7 : Sum  Inputs=++|
  w*Lf_pu : Gain  Gain=Lt_pu
  Is_dq* : Outport  InitialOutput=0  VectorParamsAs1DForOutWhenUnconnected=off
  wires:
  Gain Corrector2/1 -> Sum7/2
  Product1/1 -> Sum5/1
  Demux2/2 -> Sum6/1
  Demux2/1 -> Sum/2
  Gain Corrector3/1 -> Sum3/1
  Demux1/2 -> Product/1, Sum7/1
  w/1 -> w*Lf_pu/1
  Sum7/1 -> Mux/2  "is_q*"
  Sum3/1 -> Mux/1  "is_d*"
  Sum5/1 -> Gain Corrector2/1
  Sum6/1 -> Sum5/2
  Demux/2 -> Sum6/2
  Mux/1 -> Is_dq*/1
  Sum2/1 -> Gain Corrector3/1
  Product/1 -> Sum2/2
  w*Lf_pu/1 -> Product/2, Product1/1
  Sum/1 -> Sum2/1
  Demux1/1 -> Product1/2, Sum3/2
  Demux/1 -> Sum/1
  Vm_dq*/1 -> Demux/1
  Ig_dq/1 -> Demux1/1
  vg_dq/1 -> Demux2/1

== system Open_Loop_No_PLL/GFM_VC IDEAL_VSC1/Control loops/TVI/dq to phasor ==
  dq_mes : Inport
  Demux : Demux  Outputs=2
      settings: DisplayOption=none
  Sqrt : Sqrt  SaturateOnIntegerOverflow=on
  Sum4 : Sum  Inputs=|++  InputSameDT=on  SaturateOnIntegerOverflow=on  OutDataTypeStr=Inherit: Same as first input
  Vrdird : Product  InputSameDT=on  RndMeth=Zero  SaturateOnIntegerOverflow=on  OutDataTypeStr=Inherit: Same as first input
  Vrqirq : Product  InputSameDT=on  RndMeth=Zero  SaturateOnIntegerOverflow=on  OutDataTypeStr=Inherit: Same as first input
  rms : Outport  VectorParamsAs1DForOutWhenUnconnected=off
  wires:
  Sqrt/1 -> rms/1
  dq_mes/1 -> Demux/1
  Demux/1 -> Vrdird/1, Vrdird/2
  Demux/2 -> Vrqirq/1, Vrqirq/2
  Vrdird/1 -> Sum4/1
  Vrqirq/1 -> Sum4/2
  Sum4/1 -> Sqrt/1

== system Open_Loop_No_PLL/GFM_VC IDEAL_VSC1/Control loops/Transient Damping Resistance/Filter w_LF ==
  e : Inport
  1/T_LP : Gain  Gain=W_TVR  SaturateOnIntegerOverflow=on  OutDataTypeStr=Inherit: Same as input  ParamDataTypeStr=Inherit: Same as input
  Integrator : Integrator  InitialConditionSource=external  InitialCondition=[VSC01_id0*0.04]
  Sum1 : Sum  Inputs=|+-  InputSameDT=on  SaturateOnIntegerOverflow=on  OutDataTypeStr=Inherit: Same as first input
  s : Outport  VectorParamsAs1DForOutWhenUnconnected=off
  wires:
  Sum1/1 -> 1/T_LP/1
  1/T_LP/1 -> Integrator/1
  Integrator/1 -> Sum1/2, s/1
  e/1 -> Integrator/2, Sum1/1
